simulink model "ATTACC"  (R2021a)
settings: Solver=VariableStepAuto  StartTime=0.0  StopTime=14.42  RelTol=1e-3
model workspace: external: MAT-File C:\Users\Documents\ICLR\control system design\rocket_workspace.mat (data not in the file)
libraries: SignalEditorBlockLib x4, pid_lib x1
settings Model: Creator=hayleywong  LastModifiedBy=user
settings SolverCC: AlgebraicLoopSolver=TrustRegion
settings DebuggingCC: SFMachineParentedDataDiag=warning

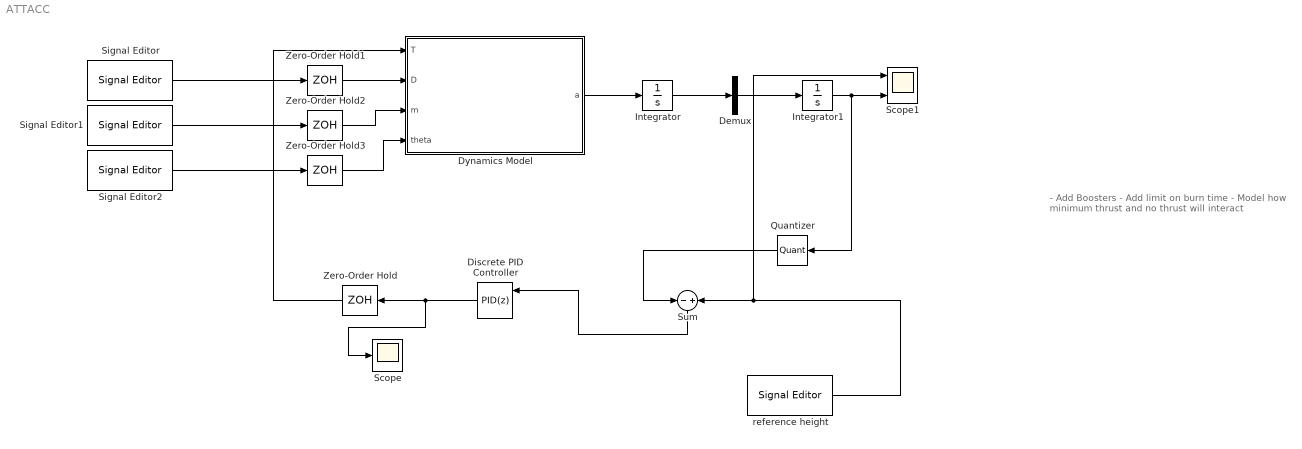
== system ATTACC ==
  note: - Add Boosters
      | - Add limit on burn time
      | - Model how minimum thrust and no thrust will interact
  Demux : Demux  Outputs=1
  Discrete PID Controller : pid_lib/PID Controller  Controller=PID  Form=Parallel  TimeDomain=Discrete-time  UseExternalTs=off  SampleTime=-1  IntegratorMethod=Forward Euler  FilterMethod=Forward Euler  ControllerParametersSource=internal  P=10  I=2  D=115  UseFilter=off  N=100  TunerSelectOption=Transfer Function Based (PID Tuner App)  InitialConditionSource=external  InitialConditionForIntegrator=0  InitialConditionForFilter=0  DifferentiatorICPrevScaledInput=0  ExternalReset=none  TrackingMode=off  Kt=1  LimitOutput=on  SatLimitsSource=internal  UpperSaturationLimit=1800  LowerSaturationLimit=900  LinearizeAsGain=off  AntiWindupMode=none  Kb=1  POutMin=[]  POutMax=[]  IOutMin=[]  IOutMax=[]  DOutMin=[]  DOutMax=[]  NOutMin=[]  NOutMax=[]  SumOutMin=[]  SumOutMax=[]  SaturationOutMin=[]  SaturationOutMax=[]  PParamMin=[]  PParamMax=[]  IParamMin=[]  IParamMax=[]  DParamMin=[]  DParamMax=[]  NParamMin=[]  NParamMax=[]  KbParamMin=[]  KbParamMax=[]  KtParamMin=[]  KtParamMax=[]  KbOutMin=[]  KbOutMax=[]  KtOutMin=[]  KtOutMax=[]  IntegratorOutMin=[]  IntegratorOutMax=[]  FilterOutMin=[]  FilterOutMax=[]  SumI1OutMin=[]  SumI1OutMax=[]  SumI2OutMin=[]  SumI2OutMax=[]  SumI3OutMin=[]  SumI3OutMax=[]  SumI4OutMin=[]  SumI4OutMax=[]  SumDOutMin=[]  SumDOutMax=[]  DifferentiatorOutMin=[]  DifferentiatorOutMax=[]  FilterDiffOutCoefMin=[]  FilterDiffOutCoefMax=[]  ReciprocalOutMin=[]  ReciprocalOutMax=[]  SumDenOutMin=[]  SumDenOutMax=[]  SumNumOutMin=[]  SumNumOutMax=[]  DivideOutMin=[]  DivideOutMax=[]  UdiffTsProdOutMin=[]  UdiffTsProdOutMax=[]  NTsProdOutMin=[]  NTsProdOutMax=[]  UintegralTsProdOutMin=[]  UintegralTsProdOutMax=[]  UngainTsProdOutMin=[]  UngainTsProdOutMax=[]  IntegratorContinuousStateAttributes=''  IntegratorStateMustResolveToSignalObject=off  IntegratorRTWStateStorageClass=Auto  FilterContinuousStateAttributes=''  FilterStateMustResolveToSignalObject=off  FilterRTWStateStorageClass=Auto  ParallelPVariant=InternalParameters  IdealPVariant=Disabled  IVariant=InternalParameters  DVariant=InternalParameters  IntegratorVariant=Discrete  SatVariant=Enabled  AWVariant=Passthrough  PCopyVariant=Disabled  TRVariant=Disabled  FdbkBlocksVariant=Forward  IdealPFdbkVariant=Disabled  SatFdbkVariant=Disabled  DerivativeFilterVariant=Differentiator  NVariant=Passthrough  NCopyVariant=Disabled_SignalSpec  FilterICVariant=ExternalICs  IntegratorICVariant=ExternalICs  ExternalResetVariant=Disabled  TRSumVariant=Passthrough  SumFdbkVariant=Disabled  SumVariant=Sum_PID  TsampFilterVariant=InternalTs  TsampNgainVariant=Passthrough  TsampIntegralVariant=Passthrough  ExternalSaturationOutDataTypeStr=Inherit: Same as second input
  Dynamics Model : MATLAB Function  TreatAsAtomicUnit=on
  Integrator : Integrator
  Integrator1 : Integrator
  Quantizer : Quantizer
  Scope : Scope
  Scope1 : Scope  NumInputPorts=2
  Signal Editor : SignalEditorBlockLib/Signal Editor  FileName=C:\Users\user\OneDrive - Imperial College London\Documents\ICLR\control system design\OneDrive_1_5-25-2021\drag.mat  ActiveScenario=untitled  ActiveSignal=drag_timeseries  IsBus=off  OutputBusObjectStr=Bus: BusObject  SampleTime=0  Interpolate=off  ZeroCross=off  OutputAfterFinalValue=Setting to zero  Unit=inherit  PreserveSignalName=on
  Signal Editor1 : SignalEditorBlockLib/Signal Editor  FileName=C:\Users\user\OneDrive - Imperial College London\Documents\ICLR\control system design\OneDrive_1_5-25-2021\Mass.mat  ActiveScenario=untitled  ActiveSignal=mass_timeseries  IsBus=off  OutputBusObjectStr=Bus: BusObject  SampleTime=0  Interpolate=off  ZeroCross=off  OutputAfterFinalValue=Setting to zero  Unit=inherit  PreserveSignalName=on
  Signal Editor2 : SignalEditorBlockLib/Signal Editor  FileName=C:\Users\user\OneDrive - Imperial College London\Documents\ICLR\control system design\OneDrive_1_5-25-2021\flight_angle.mat  ActiveScenario=untitled  ActiveSignal=theta_timeseries  IsBus=off  OutputBusObjectStr=Bus: BusObject  SampleTime=0  Interpolate=off  ZeroCross=off  OutputAfterFinalValue=Setting to zero  Unit=inherit  PreserveSignalName=on
  Sum : Sum  Inputs=-+
  Zero-Order Hold{,1..3} (4 alike) : ZeroOrderHold  SampleTime=-1
  reference height : SignalEditorBlockLib/Signal Editor  FileName=C:\Users\user\OneDrive - Imperial College London\Documents\ICLR\control system design\OneDrive_1_5-25-2021\altitude.mat  ActiveScenario=untitled  ActiveSignal=altitude_series  IsBus=off  OutputBusObjectStr=Bus: BusObject  SampleTime=0  Interpolate=off  ZeroCross=off  OutputAfterFinalValue=Setting to zero  Unit=inherit  PreserveSignalName=on
  wires:
  Dynamics Model/1(a) -> Integrator/1
  Integrator/1 -> Demux/1
  Demux/1 -> Integrator1/1
  Signal Editor/1 -> Zero-Order Hold1/1
  Signal Editor1/1 -> Zero-Order Hold2/1
  Signal Editor2/1 -> Zero-Order Hold3/1
  Integrator1/1 -> Quantizer/1, Scope1/2
  reference height/1 -> Sum/2, Scope1/1
  Sum/1 -> Discrete PID Controller/1
  Zero-Order Hold1/1 -> Dynamics Model/2(D)
  Zero-Order Hold2/1 -> Dynamics Model/3(m)
  Zero-Order Hold3/1 -> Dynamics Model/4(theta)
  Discrete PID Controller/1 -> Zero-Order Hold/1, Scope/1
  Quantizer/1 -> Sum/1
  Zero-Order Hold/1 -> Dynamics Model/1(T)

== matlab function ATTACC/Dynamics Model ==
  data: a output; T input; D input; m input; theta input
function a = dynamics(T,D,m,theta)

g = 9.81;

a = (1/m)*(T*sin(theta)-D*sin(theta)-m*g);
return
